simulink model "MotorControl"  (R2020a)
settings: Solver=FixedStepAuto  StartTime=0.0  StopTime=10.0  FixedStep=0.001  RelTol=1e-3  EnableMultiTasking=on
libraries: arduinolib x6, simulink x2, sldrtlib x1, arduinosensorlib x1
settings Model: SimulationMode=external  SILPILModeSetting=veronly  EnablePacing=on  ExtModeTrigDuration=2  Creator=InFla  LastModifiedBy=InFla
settings SolverCC: AutoInsertRateTranBlk=on
settings OptimizationCC: EnhancedBackFolding=on  PassReuseOutputArgsAs=Individual arguments  ZeroExternalMemoryAtStartup=off  ZeroInternalMemoryAtStartup=off  MaxStackSize=64  OptimizeBlockOrder=speed  DifferentSizesBufferReuse=on  EfficientTunableParamExpr=on
settings DebuggingCC: ParameterTunabilityLossMsg=error
settings HardwareCC: ProdBitPerInt=16  ProdBitPerPointer=16  ProdBitPerSizeT=16  ProdBitPerPtrDiffT=16  ProdLargestAtomicFloat=None  ProdWordSize=8  ProdHWDeviceType=Atmel->AVR  UseEmbeddedCoderFeatures=off  UseSimulinkCoderFeatures=off
settings SFSimCC: MATLABDynamicMemAlloc=off
settings RTWCC: SystemTargetFile=ert.tlc  HardwareBoard=Arduino Uno  TLCOptions=-aInlineSetEventsForThisBaseRateFcn=TLC_FALSE -aSuppressMultiTaskScheduler=TLC_FALSE -aRateBasedStepFcn=1  TemplateMakefile=ert_default_tmf  RTWVerbose=off  Toolchain=Arduino AVR  BuildConfiguration=Faster Runs
settings CodeAppCC: ForceParamTrailComments=on  OperatorAnnotations=on  SimulinkDataObjDesc=on  SFDataObjDesc=on  MangleLength=10  InsertBlockDesc=on
settings ERTTargetCC: SupportContinuousTime=on  SupportNonInlinedSFcns=on  SupportVariableSizeSignals=on  ExtMode=on  ExtModeStaticAllocSize=250  ExtModeMexArgs='127.0.0.1' 0 17725  ERTSrcFileBannerTemplate=codertarget_code_template.cgt  ERTHdrFileBannerTemplate=codertarget_code_template.cgt  ERTDataSrcFileTemplate=codertarget_code_template.cgt  ERTDataHdrFileTemplate=codertarget_code_template.cgt

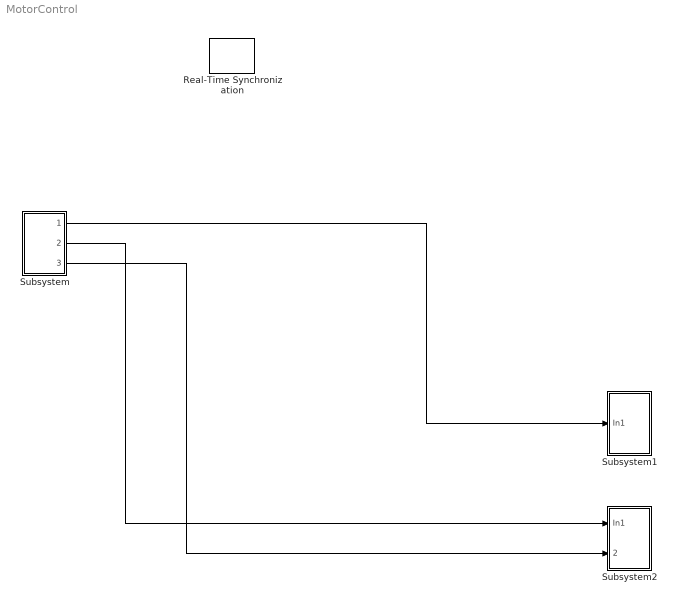
== system MotorControl ==
  Real-Time Synchronization : sldrtlib/Real-Time Synchronization  SampleTime=0.05  MaxMissedTicks=10  ShowMissedTicks=off  YieldWhenWaiting=off
  Subsystem : Subsystem
  Subsystem1 : Subsystem
  Subsystem2 : Subsystem
  wires:
  Subsystem/1(Output) -> Subsystem1/1(In1)
  Subsystem/2(Output1) -> Subsystem2/1(In1)
  Subsystem/3(Output2) -> Subsystem2/2(Output2)

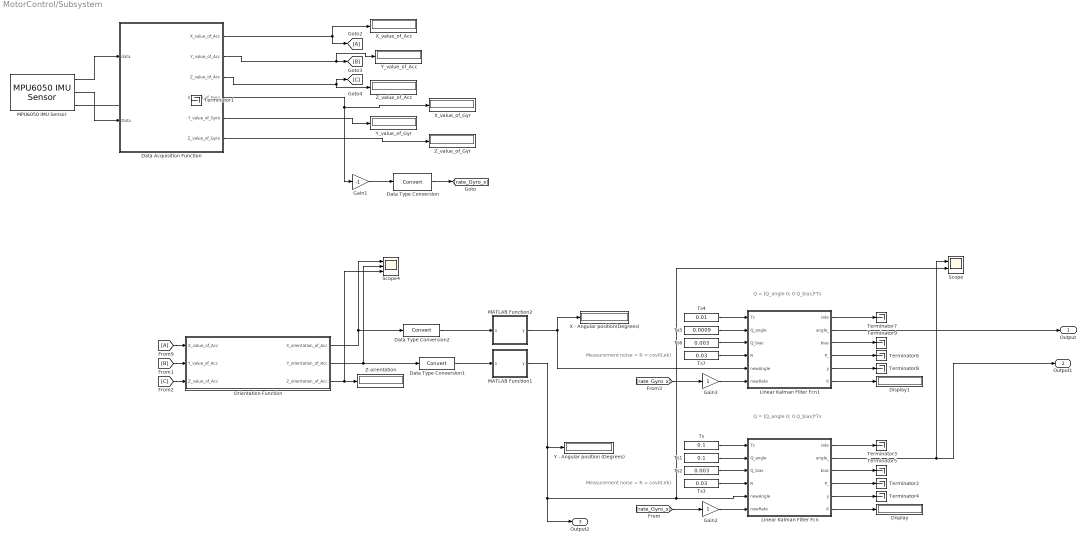
== system MotorControl/Subsystem ==
  note: Q = [Q_angle 0; 0 Q_bias]*Ts
  note: Q = [Q_angle 0; 0 Q_bias]*Ts
  note: Measurement noise = R = cov(0,ek)
  note: Measurement noise = R = cov(0,ek)
  Data Acquisition Function : MATLAB Function  TreatAsAtomicUnit=on
  Data Type Conversion : DataTypeConversion
  Data Type Conversion1 : DataTypeConversion
  Data Type Conversion2 : DataTypeConversion
  Display : Display
  Display1 : Display
  Gain1 : Gain  Gain=-1
  Gain2 : Gain
  Gain3 : Gain
  Linear Kalman Filter Fcn : MATLAB Function  TreatAsAtomicUnit=on
  Linear Kalman Filter Fcn1 : MATLAB Function  TreatAsAtomicUnit=on
  MATLAB Function1 : MATLAB Function  TreatAsAtomicUnit=on
  MATLAB Function2 : MATLAB Function  TreatAsAtomicUnit=on
  MPU6050 IMU Sensor : arduinosensorlib/MPU6050 IMU Sensor  SlaveAddress=0x68  Accel=on  AngularRate=on  Temperature=off  Status=on  EulerAngles=off  Quat=off  AccelRange=2G  GyroRange=250 dps  DmpOdr=200 Hz  Dlpf=Accelerometer: 184Hz, Gyroscope: 188Hz  SampleTime=0.05
      settings: SourceProductBaseCode=ARDUINO
  Orientation Function : MATLAB Function  TreatAsAtomicUnit=on
  Scope : Scope  NumInputPorts=2
  Scope4 : Scope  NumInputPorts=3
  Terminator{1..9} (9 alike) : Terminator
  Ts : Constant  Value=0.1
  Ts1 : Constant  Value=0.1
  Ts2 : Constant  Value=0.003
  Ts3 : Constant  Value=0.03
  Ts4 : Constant  Value=0.01
  Ts5 : Constant  Value=0.0009
  Ts6 : Constant  Value=0.003
  Ts7 : Constant  Value=0.03
  X - Angular position(Degrees) : Display
  X_value_of_Acc : Display
      settings: Format=bank
  X_value_of_Gyr : Display
      settings: Format=bank
  Y - Angular position (Degrees) : Display
  Y_value_of_Acc : Display
      settings: Format=bank
  Y_value_of_Gyr : Display
      settings: Format=bank
  Z-orientation : Display
      settings: Format=bank
  Z_value_of_Acc : Display
      settings: Format=bank
  Z_value_of_Gyr : Display
      settings: Format=bank
  Output : Outport
  Output1 : Outport  Port=2
  Output2 : Outport  Port=3
  wires:
  Data Acquisition Function/4(X_value_of_Gyro) -> X_value_of_Gyr/1, Gain1/1
  Linear Kalman Filter Fcn/1(rate) -> Terminator3/1
  [rate_Gyro_x] -> Gain2/1
  Linear Kalman Filter Fcn/2(angle_) -> Scope/1, Output1/1
  Linear Kalman Filter Fcn/3(bias) -> Terminator5/1
  Linear Kalman Filter Fcn1/1(rate) -> Terminator7/1
  Ts5/1 -> Linear Kalman Filter Fcn1/2(Q_angle)
  Ts6/1 -> Linear Kalman Filter Fcn1/3(Q_bias)
  Orientation Function/1(X_orientation_of_Acc) -> Scope4/1, Data Type Conversion2/1
  Data Type Conversion1/1 -> MATLAB Function1/1(u)
  [rate_Gyro_x] -> Gain3/1
  MATLAB Function1/1(y) -> Output2/1, Scope/2, Linear Kalman Filter Fcn/5(newAngle), Y - Angular position (Degrees)/1
  Orientation Function/2(Y_orientation_of_Acc) -> Data Type Conversion1/1, Scope4/2
  MATLAB Function2/1(y) -> Linear Kalman Filter Fcn1/5(newAngle), X - Angular position(Degrees)/1
  Data Type Conversion2/1 -> MATLAB Function2/1(u)
  Linear Kalman Filter Fcn1/2(angle_) -> Output/1
  MPU6050 IMU Sensor/3 -> Terminator1/1
  Ts2/1 -> Linear Kalman Filter Fcn/3(Q_bias)
  Data Acquisition Function/6(Z_value_of_Gyro) -> Z_value_of_Gyr/1
  Data Acquisition Function/3(Z_value_of_Acc) -> Z_value_of_Acc/1, [C]
  [C] -> Orientation Function/3(Z_value_of_Acc)
  Linear Kalman Filter Fcn/4(P_) -> Terminator2/1
  Linear Kalman Filter Fcn1/6(K) -> Display1/1
  Gain2/1 -> Linear Kalman Filter Fcn/6(newRate)
  Gain3/1 -> Linear Kalman Filter Fcn1/6(newRate)
  Data Type Conversion/1 -> [rate_Gyro_x]
  [A] -> Orientation Function/1(X_value_of_Acc)
  [B] -> Orientation Function/2(Y_value_of_Acc)
  Ts3/1 -> Linear Kalman Filter Fcn/4(R)
  Data Acquisition Function/2(Y_value_of_Acc) -> Y_value_of_Acc/1, [B]
  Ts7/1 -> Linear Kalman Filter Fcn1/4(R)
  Data Acquisition Function/1(X_value_of_Acc) -> [A], X_value_of_Acc/1
  Linear Kalman Filter Fcn1/4(P_) -> Terminator6/1
  Ts4/1 -> Linear Kalman Filter Fcn1/1(Ts)
  Linear Kalman Filter Fcn1/3(bias) -> Terminator9/1
  Linear Kalman Filter Fcn/6(K) -> Display/1
  Linear Kalman Filter Fcn/5(y) -> Terminator4/1
  MPU6050 IMU Sensor/2 -> Data Acquisition Function/2(Data)
  Data Acquisition Function/5(Y_value_of_Gyro) -> Y_value_of_Gyr/1
  Orientation Function/3(Z_orientation_of_Acc) -> Scope4/3, Z-orientation/1
  Linear Kalman Filter Fcn1/5(y) -> Terminator8/1
  Gain1/1 -> Data Type Conversion/1
  Ts/1 -> Linear Kalman Filter Fcn/1(Ts)
  MPU6050 IMU Sensor/1 -> Data Acquisition Function/1(data)
  Ts1/1 -> Linear Kalman Filter Fcn/2(Q_angle)

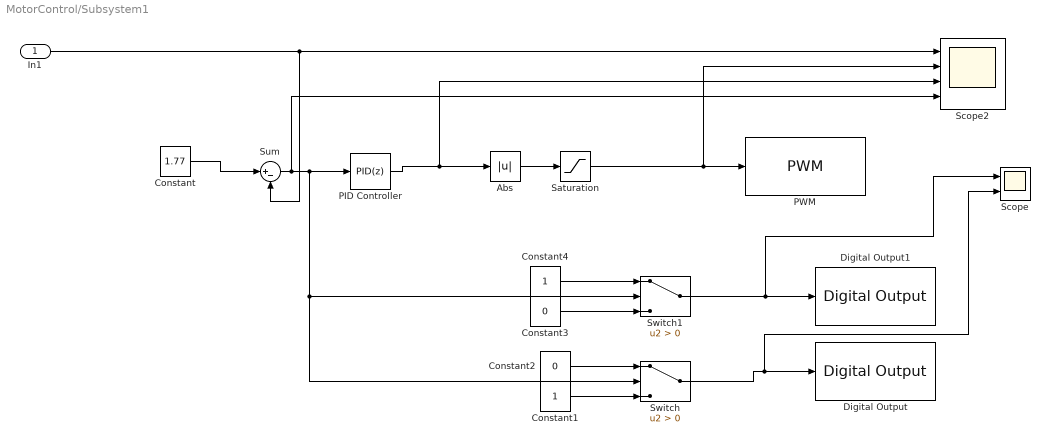
== system MotorControl/Subsystem1 ==
  In1 : Inport
  Abs : Abs
  Constant : Constant  Value=1.77
  Constant1 : Constant
  Constant2 : Constant  Value=0
  Constant3 : Constant  Value=0
  Constant4 : Constant
  Digital Output : arduinolib/Digital Output  pinNumber=8  Direction=output  blockPlatform=arduino
  Digital Output1 : arduinolib/Digital Output  pinNumber=7  Direction=output  blockPlatform=arduino
  PID Controller : simulink/Continuous/PID Controller  Controller=PID  Form=Parallel  TimeDomain=Discrete-time  UseExternalTs=off  SampleTime=0.01  IntegratorMethod=Forward Euler  FilterMethod=Forward Euler  ControllerParametersSource=internal  P=1  I=0.05  D=1  UseFilter=on  N=100  TunerSelectOption=Transfer Function Based (PID Tuner App)  InitialConditionSource=internal  InitialConditionForIntegrator=0  InitialConditionForFilter=0  DifferentiatorICPrevScaledInput=0  ExternalReset=none  TrackingMode=off  Kt=1  LimitOutput=off  UpperSaturationLimit=inf  LowerSaturationLimit=-inf  LinearizeAsGain=on  AntiWindupMode=none  Kb=1  POutMin=[]  POutMax=[]  IOutMin=[]  IOutMax=[]  DOutMin=[]  DOutMax=[]  NOutMin=[]  NOutMax=[]  SumOutMin=[]  SumOutMax=[]  SaturationOutMin=[]  SaturationOutMax=[]  PParamMin=[]  PParamMax=[]  IParamMin=[]  IParamMax=[]  DParamMin=[]  DParamMax=[]  NParamMin=[]  NParamMax=[]  KbParamMin=[]  KbParamMax=[]  KtParamMin=[]  KtParamMax=[]  KbOutMin=[]  KbOutMax=[]  KtOutMin=[]  KtOutMax=[]  IntegratorOutMin=[]  IntegratorOutMax=[]  FilterOutMin=[]  FilterOutMax=[]  SumI1OutMin=[]  SumI1OutMax=[]  SumI2OutMin=[]  SumI2OutMax=[]  SumI3OutMin=[]  SumI3OutMax=[]  SumI4OutMin=[]  SumI4OutMax=[]  SumDOutMin=[]  SumDOutMax=[]  DifferentiatorOutMin=[]  DifferentiatorOutMax=[]  FilterDiffOutCoefMin=[]  FilterDiffOutCoefMax=[]  ReciprocalOutMin=[]  ReciprocalOutMax=[]  SumDenOutMin=[]  SumDenOutMax=[]  SumNumOutMin=[]  SumNumOutMax=[]  DivideOutMin=[]  DivideOutMax=[]  UdiffTsProdOutMin=[]  UdiffTsProdOutMax=[]  NTsProdOutMin=[]  NTsProdOutMax=[]  UintegralTsProdOutMin=[]  UintegralTsProdOutMax=[]  UngainTsProdOutMin=[]  UngainTsProdOutMax=[]  IntegratorContinuousStateAttributes=''  IntegratorStateMustResolveToSignalObject=off  IntegratorRTWStateStorageClass=Auto  FilterContinuousStateAttributes=''  FilterStateMustResolveToSignalObject=off  FilterRTWStateStorageClass=Auto  ParallelPVariant=InternalParameters  IdealPVariant=Disabled  IVariant=InternalParameters  DVariant=InternalParameters  IntegratorVariant=Discrete  SatVariant=Disabled  AWVariant=Passthrough  PCopyVariant=Disabled  TRVariant=Disabled  FdbkBlocksVariant=Forward  IdealPFdbkVariant=Disabled  SatFdbkVariant=Disabled  DerivativeFilterVariant=ForwardEulerFilter  NVariant=InternalParameters  NCopyVariant=Disabled  FilterICVariant=InternalICsFilter  IntegratorICVariant=InternalICs  ExternalResetVariant=Disabled  TRSumVariant=Passthrough  SumFdbkVariant=Disabled  SumVariant=Sum_PID  TsampFilterVariant=InternalTs  TsampNgainVariant=Passthrough  TsampIntegralVariant=Passthrough
  PWM : arduinolib/PWM  pinNumber=9  frequencyType=Default  desiredFrequency=490.2  achievableFrequency=490.2
  Saturation : Saturate  UpperLimit=255  LowerLimit=0
  Scope : Scope  NumInputPorts=2
  Scope2 : Scope  NumInputPorts=4
  Sum : Sum  Inputs=|+-
  Switch : Switch  Criteria=u2 > Threshold
  Switch1 : Switch  Criteria=u2 > Threshold
  wires:
  Constant2/1 -> Switch/1
  Constant/1 -> Sum/1
  Switch/1 -> Scope/2, Digital Output/1
  Switch1/1 -> Scope/1, Digital Output1/1
  Abs/1 -> Saturation/1
  In1/1 -> Sum/2, Scope2/1
  Saturation/1 -> PWM/1, Scope2/2
  Constant4/1 -> Switch1/1
  Sum/1 -> Scope2/4, Switch1/2, Switch/2, PID Controller/1
  Constant3/1 -> Switch1/3
  Constant1/1 -> Switch/3
  PID Controller/1 -> Scope2/3, Abs/1

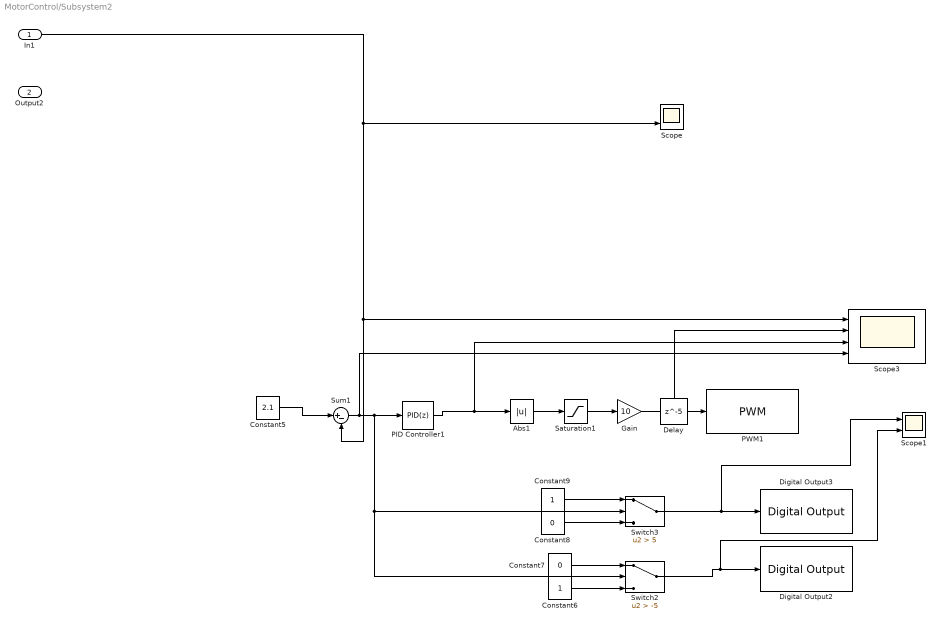
== system MotorControl/Subsystem2 ==
  In1 : Inport
  Output2 : Inport  Port=2
  Abs1 : Abs
  Constant5 : Constant  Value=2.1
  Constant6 : Constant
  Constant7 : Constant  Value=0
  Constant8 : Constant  Value=0
  Constant9 : Constant
  Delay : Delay  DelayLength=5
  Digital Output2 : arduinolib/Digital Output  pinNumber=4  Direction=output  blockPlatform=arduino
  Digital Output3 : arduinolib/Digital Output  pinNumber=2  Direction=output  blockPlatform=arduino
  Gain : Gain  Gain=10
  PID Controller1 : simulink/Continuous/PID Controller  Controller=PID  Form=Parallel  TimeDomain=Discrete-time  UseExternalTs=off  SampleTime=0.01  IntegratorMethod=Forward Euler  FilterMethod=Forward Euler  ControllerParametersSource=internal  P=1  I=1  D=0  UseFilter=on  N=100  TunerSelectOption=Transfer Function Based (PID Tuner App)  InitialConditionSource=internal  InitialConditionForIntegrator=0  InitialConditionForFilter=0  DifferentiatorICPrevScaledInput=0  ExternalReset=none  TrackingMode=off  Kt=1  LimitOutput=off  UpperSaturationLimit=inf  LowerSaturationLimit=-inf  LinearizeAsGain=on  AntiWindupMode=none  Kb=1  POutMin=[]  POutMax=[]  IOutMin=[]  IOutMax=[]  DOutMin=[]  DOutMax=[]  NOutMin=[]  NOutMax=[]  SumOutMin=[]  SumOutMax=[]  SaturationOutMin=[]  SaturationOutMax=[]  PParamMin=[]  PParamMax=[]  IParamMin=[]  IParamMax=[]  DParamMin=[]  DParamMax=[]  NParamMin=[]  NParamMax=[]  KbParamMin=[]  KbParamMax=[]  KtParamMin=[]  KtParamMax=[]  KbOutMin=[]  KbOutMax=[]  KtOutMin=[]  KtOutMax=[]  IntegratorOutMin=[]  IntegratorOutMax=[]  FilterOutMin=[]  FilterOutMax=[]  SumI1OutMin=[]  SumI1OutMax=[]  SumI2OutMin=[]  SumI2OutMax=[]  SumI3OutMin=[]  SumI3OutMax=[]  SumI4OutMin=[]  SumI4OutMax=[]  SumDOutMin=[]  SumDOutMax=[]  DifferentiatorOutMin=[]  DifferentiatorOutMax=[]  FilterDiffOutCoefMin=[]  FilterDiffOutCoefMax=[]  ReciprocalOutMin=[]  ReciprocalOutMax=[]  SumDenOutMin=[]  SumDenOutMax=[]  SumNumOutMin=[]  SumNumOutMax=[]  DivideOutMin=[]  DivideOutMax=[]  UdiffTsProdOutMin=[]  UdiffTsProdOutMax=[]  NTsProdOutMin=[]  NTsProdOutMax=[]  UintegralTsProdOutMin=[]  UintegralTsProdOutMax=[]  UngainTsProdOutMin=[]  UngainTsProdOutMax=[]  IntegratorContinuousStateAttributes=''  IntegratorStateMustResolveToSignalObject=off  IntegratorRTWStateStorageClass=Auto  FilterContinuousStateAttributes=''  FilterStateMustResolveToSignalObject=off  FilterRTWStateStorageClass=Auto  ParallelPVariant=InternalParameters  IdealPVariant=Disabled  IVariant=InternalParameters  DVariant=InternalParameters  IntegratorVariant=Discrete  SatVariant=Disabled  AWVariant=Passthrough  PCopyVariant=Disabled  TRVariant=Disabled  FdbkBlocksVariant=Forward  IdealPFdbkVariant=Disabled  SatFdbkVariant=Disabled  DerivativeFilterVariant=ForwardEulerFilter  NVariant=InternalParameters  NCopyVariant=Disabled  FilterICVariant=InternalICsFilter  IntegratorICVariant=InternalICs  ExternalResetVariant=Disabled  TRSumVariant=Passthrough  SumFdbkVariant=Disabled  SumVariant=Sum_PID  TsampFilterVariant=InternalTs  TsampNgainVariant=Passthrough  TsampIntegralVariant=Passthrough
  PWM1 : arduinolib/PWM  pinNumber=3  frequencyType=Default  desiredFrequency=490.2  achievableFrequency=490.2
  Saturation1 : Saturate  UpperLimit=5  LowerLimit=0
  Scope : Scope  NumInputPorts=2
  Scope1 : Scope  NumInputPorts=2
  Scope3 : Scope  NumInputPorts=4
  Sum1 : Sum  Inputs=|+-
  Switch2 : Switch  Criteria=u2 > Threshold  Threshold=-5
  Switch3 : Switch  Criteria=u2 > Threshold  Threshold=5
  wires:
  Sum1/1 -> Scope3/4, Switch2/2, Switch3/2, PID Controller1/1
  Switch3/1 -> Scope1/1, Digital Output3/1
  PID Controller1/1 -> Scope3/3, Abs1/1
  Constant9/1 -> Switch3/1
  Constant7/1 -> Switch2/1
  Constant6/1 -> Switch2/3
  Constant8/1 -> Switch3/3
  In1/1 -> Sum1/2, Scope3/1, Scope/2
  Constant5/1 -> Sum1/1
  Abs1/1 -> Saturation1/1
  Switch2/1 -> Scope1/2, Digital Output2/1
  Saturation1/1 -> Gain/1
  Gain/1 -> PWM1/1, Scope3/2

== matlab function MotorControl/Subsystem/MATLAB Function1 ==
  data: u input; y output
function y = fcn(u)

if(isnan(u))
y=0;
else
y=u;
end

== matlab function MotorControl/Subsystem/Linear Kalman Filter Fcn ==
  settings: updateMethod=DISCRETE
  data: Ts input; Q_angle input; Q_bias input; R input; newAngle input; rate output; newRate input; angle_ output; bias output; P_ output; y output; K output
% Algorithm -- implimentation of Linear-Kalman filter for a 6-DOF IMU using
% a single axis for testing. A single axis consisting of both anaccelerometer
% input and gyroscope input from IMU.
% Author: RM van Rensburg
% for IMU testing purposes
% Date: 26-04-2015
% Version: 1.0,tested on Matlab R2015a

function [rate,angle_,bias,P_,y,K] = Kalmanf(Ts,...
                                             Q_angle,Q_bias,R,...
                                             newAngle,...
                                             newRate)
                      
% Process noise covariance matrix  
Q = [Q_angle 0;0 Q_bias]*Ts;
A = [1  -Ts;0  1];
C = [1 0];
bias = 0.0;

rate = newRate - bias;

persistent angle;
if isempty(angle);angle = 0;
else angle = angle + (Ts * rate); 
end
angle_= angle;
                    
persistent P;
if isempty(P);P = [0 0 ; 0 0]; 
else P = A*P*A' + Q;
end
P_=P;

S = C*P*C' + R; % Estimate error 
K = (P_*C')/S; % Kalman gain
y = newAngle - angle_; % Angle difference 
xk = angle_ + K*y;
angle_ = xk(1);
bias = xk(2);
angle = angle_;

% Update the error covariance 
I = [1 0;0 1];
P_ = (I - K*C)*P_;
% or
% Joseph form (more stable)
% P_ = (I - K*C)*P_*(I - K*C) + K*R*K';
P = P_;

return

end

== matlab function MotorControl/Subsystem/Linear Kalman Filter Fcn1 ==
  settings: updateMethod=DISCRETE
  data: Ts input; Q_angle input; Q_bias input; R input; newAngle input; rate output; newRate input; angle_ output; bias output; P_ output; y output; K output
% Algorithm -- implimentation of Linear-Kalman filter for a 6-DOF IMU using
% a single axis for testing. A single axis consisting of both anaccelerometer
% input and gyroscope input from IMU.
% Author: RM van Rensburg
% for IMU testing purposes
% Date: 26-04-2015
% Version: 1.0,tested on Matlab R2015a

function [rate,angle_,bias,P_,y,K] = Kalmanf(Ts,...
                                             Q_angle,Q_bias,R,...
                                             newAngle,...
                                             newRate)
                      
% Process noise covariance matrix  
Q = [Q_angle 0;0 Q_bias]*Ts;
A = [1  -Ts;0  1];
C = [1 0];
bias = 0.0;

rate = newRate - bias;

persistent angle;
if isempty(angle);angle = 0;
else angle = angle + (Ts * rate); 
end
angle_= angle;
                    
persistent P;
if isempty(P);P = [0 0 ; 0 0]; 
else P = A*P*A' + Q;
end
P_=P;

S = C*P*C' + R; % Estimate error 
K = (P_*C')/S; % Kalman gain
y = newAngle - angle_; % Angle difference 
xk = angle_ + K*y;
angle_ = xk(1);
bias = xk(2);
angle = angle_;

% Update the error covariance 
I = [1 0;0 1];
P_ = (I - K*C)*P_;
% or
% Joseph form (more stable)
% P_ = (I - K*C)*P_*(I - K*C) + K*R*K';
P = P_;

return

end

== matlab function MotorControl/Subsystem/Data Acquisition Function ==
  data: data input; Data input; X_value_of_Acc output; Y_value_of_Acc output; Z_value_of_Acc output; X_value_of_Gyro output; Y_value_of_Gyro output; Z_value_of_Gyro output
% Reading IMU packet bytes from Sensor Stream App 
% Author: RM van Rensburg
% Date: 26-04-2015
% Version: 1.0,tested on Matlab R2015a

function [X_value_of_Acc,Y_value_of_Acc, Z_value_of_Acc,...
          X_value_of_Gyro, Y_value_of_Gyro, Z_value_of_Gyro]...
          = fcn(data, Data)
             
% Header packet
% Header = Data(1:4);

% Accelerometer data
X_value_of_Acc = data(1,:);
Y_value_of_Acc = data(2,:);
Z_value_of_Acc = data(3,:);

% Gyroscope data
X_value_of_Gyro = Data(1,:);
Y_value_of_Gyro = Data(2,:);
Z_value_of_Gyro = Data(3,:);

% Proximity sensor
% X_value_of_Tes = typecast(uint8(Data(29:36)),'double');
% Y_value_of_Tes = typecast(uint8(Data(37:44)),'double');
% Z_value_of_Tes = typecast(uint8(Data(45:52)),'double');

== matlab function MotorControl/Subsystem/MATLAB Function2 ==
  data: u input; y output
function y = fcn(u)

if(isnan(u))
y=0;
else
y=u;
end

== matlab function MotorControl/Subsystem/Orientation Function ==
  data: X_value_of_Acc input; X_orientation_of_Acc output; Y_orientation_of_Acc output; Z_orientation_of_Acc output; Y_value_of_Acc input; Z_value_of_Acc input
% Computing orientation of tri-axial acclerometer data from IMU 
% Author: RM van Rensburg
% Date: 26-04-2015
% Version: 1.0,tested on Matlab R2015a

function [X_orientation_of_Acc,...
          Y_orientation_of_Acc,...
          Z_orientation_of_Acc]...
          = OrientationFcn(X_value_of_Acc,Y_value_of_Acc,Z_value_of_Acc)
     
      
% Using x and y from accelerometer (g-forces), calculate x and y angles
% Data directly obtained from IMU
% Using the following formulae
% Ax = arctan{X/sqrt(Y*Y + Z*Z)}
% Ay = arctan{Y/sqrt(X*X + Z*Z)}

% Computing the X*X, Y*Y, Z*Z
X2 = power(X_value_of_Acc,2);
Y2 = power(Y_value_of_Acc,2);
Z2 = power(Z_value_of_Acc,2);

% x-axis angle
result = sqrt(Y2 + Z2);
result = X_value_of_Acc / result;
x_angle_rad = atan(result);
X_orientation_of_Acc = (x_angle_rad * 180) / pi;

% y-axis angle
result = sqrt(X2 + Z2);
result = Y_value_of_Acc / result;
y_angle_rad = atan(result);
Y_orientation_of_Acc = (y_angle_rad * 180) / pi;

% z-axis angle
result = sqrt(Y2 + X2);
result = Z_value_of_Acc / result;
z_angle_rad = atan(result);
Z_orientation_of_Acc = (z_angle_rad * 180) / pi;

end
